simulink model "ClusterControl"  (R2023b)
settings: Solver=FixedStepAuto  StartTime=0.0  StopTime=inf  RelTol=1e-3
model workspace (MAT data in the model file):
  Param = Simulink.Parameter
  Param.Value = 1
  Param.DataType = 'auto'
  Param.Complexity = 'real'
  Param.Dimensions = [1 1]
  RPM_Gain = Simulink.Parameter
  RPM_Gain.Value = 2
  RPM_Gain.DataType = 'int32'
  RPM_Gain.Complexity = 'real'
  RPM_Gain.Dimensions = [1 1]
  SharedP = Simulink.Parameter
  SharedP.Value = 2
  SharedP.DataType = 'auto'
  SharedP.Complexity = 'real'
  SharedP.Dimensions = [1 1]
Description:
  | This model is for use with QML-based GUI to be deployed on a Raspberry Pi, showing an Automotive Instrument Cluster.
  | 
  | The model's purpose is to handle the backend logic, physics and CAN data communications and offload the work from direct C++ code in Qt
settings Model: ParameterArgumentNames=Param  Creator=Joel Sadler  LastModifiedBy=joel
settings SolverCC: AlgebraicLoopSolver=TrustRegion  MaxZcPerStep=1
settings OptimizationCC: OptimizeBlockIOStorage=off  BufferReuse=off  ReuseModelBlockBuffer=off  GlobalBufferReuse=off  ExpressionFolding=off  EnableMemcpy=off  PassReuseOutputArgsAs=Individual arguments  LocalBlockOutputs=off  ZeroExternalMemoryAtStartup=off  ZeroInternalMemoryAtStartup=off  OptimizeDataStoreBuffers=off  BusAssignmentInplaceUpdate=off  OptimizationLevel=level0  OptimizationCustomize=off  EfficientTunableParamExpr=on
settings DebuggingCC: ParameterTunabilityLossMsg=error  UnconnectedInputMsg=warning  UnconnectedOutputMsg=warning  UnconnectedLineMsg=warning
settings HardwareCC: ProdBitPerLong=64  ProdLargestAtomicInteger=LongLong  ProdLargestAtomicFloat=Double  ProdLongLongMode=on  ProdHWDeviceType=ARM Compatible->ARM Cortex-A (64-bit)
settings ModelReferenceCC: EnableRefExpFcnMdlSchedulingChecks=on
settings SFSimCC: MATLABDynamicMemAlloc=off
settings RTWCC: Description=Embedded Coder  SystemTargetFile=ert.tlc  TemplateMakefile=ert_default_tmf  GenerateReport=on  RTWVerbose=off  CodeExecutionProfiling=on  CodeProfilingInstrumentation=coarse  TargetLang=C++  DLArmComputeVersion=19.05
settings CodeAppCC: ForceParamTrailComments=on  IgnoreCustomStorageClasses=off  OperatorAnnotations=on  SimulinkDataObjDesc=on  SFDataObjDesc=on  InsertBlockDesc=on
settings ERTTargetCC: TargetLangStandard=C++03 (ISO)  UtilityFuncGeneration=Shared location  GenerateSampleERTMain=on  CodeInterfacePackaging=C++ class  RootIOFormat=Structure reference  ERTCustomFileTemplate=example_file_process.tlc

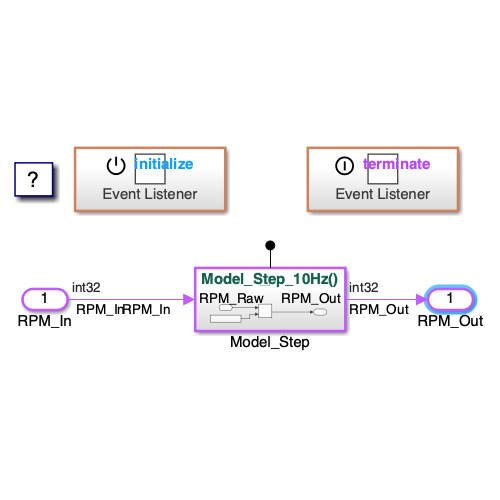
[thumbnail: Simulink's stored preview of the top-level diagram]
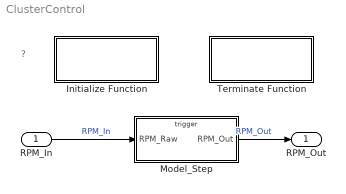
== system ClusterControl ==
  note: ?
  RPM_In : Inport  OutDataTypeStr=int32
  Initialize Function : Subsystem  TreatAsAtomicUnit=on
  Model_Step : Subsystem  TreatAsAtomicUnit=on
  Terminate Function : Subsystem  TreatAsAtomicUnit=on
  RPM_Out : Outport
  wires:
  RPM_In/1 -> Model_Step/1(RPM_Raw)  "RPM_In"
  Model_Step/1(RPM_Out) -> RPM_Out/1  "RPM_Out"

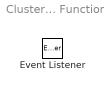
== system ClusterControl/Initialize Function ==
  Event Listener : EventListener  DisableCoverage=on  EventName=reset

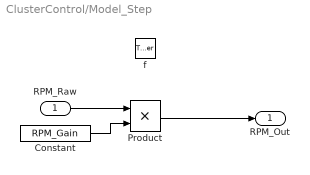
== system ClusterControl/Model_Step ==
  RPM_Raw : Inport
  f : TriggerPort  TriggerType=function-call  IsSimulinkFunction=on  FunctionName=Model_Step_10Hz  FunctionVisibility=scoped  VariantControl=(inherit)
  Constant : Constant  Value=RPM_Gain  SampleTime=-1
  Product : Product  OutDataTypeStr=Inherit: Inherit via back propagation  RndMeth=Nearest
  RPM_Out : Outport
  wires:
  RPM_Raw/1 -> Product/1
  Product/1 -> RPM_Out/1
  Constant/1 -> Product/2

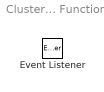
== system ClusterControl/Terminate Function ==
  Event Listener : EventListener  DisableCoverage=on  EventType=Terminate  EventName=reset
